simulink model "es2_sim"  (R2023b)
settings: Solver=VariableStepAuto  StartTime=0.0  StopTime=500  RelTol=1e-3
undefined symbols (not defined in the file or in its folder): x0
settings Model: Creator=claudio  LastModifiedBy=stefa
settings OptimizationCC: ReuseModelBlockBuffer=off

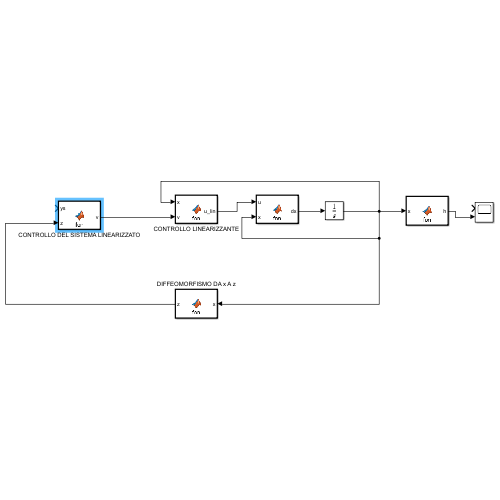
[thumbnail: Simulink's stored preview of the top-level diagram]
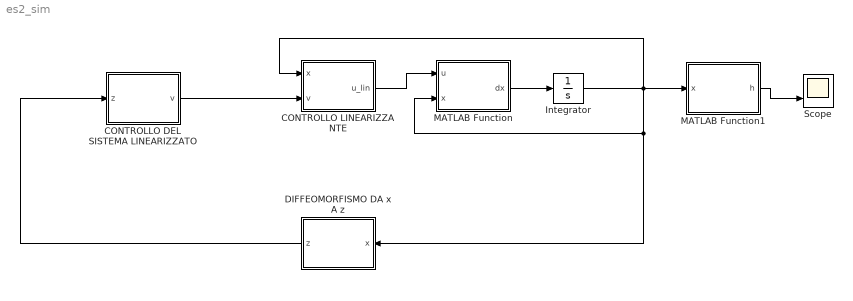
== system es2_sim ==
  CONTROLLO DEL SISTEMA LINEARIZZATO : MATLAB Function  TreatAsAtomicUnit=on
  CONTROLLO LINEARIZZANTE : MATLAB Function  TreatAsAtomicUnit=on
  DIFFEOMORFISMO DA x A z : MATLAB Function  TreatAsAtomicUnit=on
  Integrator : Integrator  InitialCondition=x0'
  MATLAB Function : MATLAB Function  TreatAsAtomicUnit=on
  MATLAB Function1 : MATLAB Function  TreatAsAtomicUnit=on
  Scope : Scope  NumInputPorts=2
  wires:
  MATLAB Function/1(dx) -> Integrator/1
  Integrator/1 -> MATLAB Function1/1(x), DIFFEOMORFISMO DA x A z/1(x), MATLAB Function/2(x), CONTROLLO LINEARIZZANTE/1(x)
  CONTROLLO LINEARIZZANTE/1(u_lin) -> MATLAB Function/1(u)
  CONTROLLO DEL SISTEMA LINEARIZZATO/1(v) -> CONTROLLO LINEARIZZANTE/2(v)
  DIFFEOMORFISMO DA x A z/1(z) -> CONTROLLO DEL SISTEMA LINEARIZZATO/1(z)
  MATLAB Function1/1(h) -> Scope/2

== matlab function es2_sim/MATLAB Function ==
  data: u input; dx output; x input
function dx = fcn(u,x)
b=0.1;
a1=0.02; %
a2=0.001; %
k=100; %

%definizione di variabili di tipo simbolico 
%scrivo dx/dt=f(x,u) (in questo caso u=d)
A=x(1);
P=x(2);
dx=[A*(1-A/k)-P*A*a1;-b*P+A*P*a2+u];

== matlab function es2_sim/CONTROLLO DEL SISTEMA LINEARIZZATO ==
  data: z input; v output
function v = fcn(z)
z1=z(1);
z2=z(2);
K=[ 1.0000   10.1000]; % risultato del comando place
v=-K(1)*z1-K(2)*z2;

== matlab function es2_sim/DIFFEOMORFISMO DA x A z ==
  data: x input; z output
function z = fcn(x)
x1=x(1);
x2=x(2);
z=[x1;- x1*(x1/100 - 1) - (x1*x2)/50];

== matlab function es2_sim/MATLAB Function1 ==
  data: h output; x input
function h = fcn(x)
h=x(1);

== matlab function es2_sim/CONTROLLO LINEARIZZANTE ==
  data: x input; v input; u_lin output
function u_lin = fcn(x,v)
x1=x(1);
x2=x(2);
u_lin=(10*x1^3 + 29*x1^2*x2 - 1500*x1^2 + 20*x1*x2^2 - 1900*x1*x2 + 50000*x1 - 50000*v)/(1000*x1)
